simulink model "AlmostWorking_TheNotebookEdition"  (R2024b)
settings: Solver=FixedStepAuto  StartTime=0.0  StopTime=inf  RelTol=1e-3  EnableMultiTasking=on
libraries: vexarmcortexlib x20, vexcommonlib x2
settings Model: Creator=ierdn  LastModifiedBy=ierdn
settings DataIOCC: LimitDataPoints=on  SignalLoggingSaveFormat=ModelDataLogs  ReturnWorkspaceOutputs=off
settings OptimizationCC: ExpressionDepthLimit=2147483647  LifeSpan=Inf  MaxStackSize=64  EfficientTunableParamExpr=on
settings DebuggingCC: UnderspecifiedInitializationDetection=Classic  MergeDetectMultiDrivingBlocksExec=none  InheritedTsInSrcMsg=none  FcnCallInpInsideContextMsg=warning  StateNameClashWarn=warning  SFUnexpectedBacktrackingDiag=warning  SFNoUnconditionalDefaultTransitionDiag=warning  SFExecutionAtInitializationDiag=none  ArithmeticOperatorsInVariantConditions=warning
settings HardwareCC: ProdBitPerPointer=32  ProdBitPerSizeT=32  ProdBitPerPtrDiffT=32  ProdLargestAtomicInteger=Long  ProdLargestAtomicFloat=Double  ProdIntDivRoundTo=Undefined  ProdWordSize=32  ProdHWDeviceType=ARM Compatible->ARM Cortex
settings ModelReferenceCC: EnableRefExpFcnMdlSchedulingChecks=on  PropagateSignalLabelsOutOfModel=off
settings SFSimCC: MATLABDynamicMemAlloc=off  CustomCodeUndefinedFunction=UseInterfaceOnly
settings RTWCC: Description=Embedded Coder  SystemTargetFile=ert.tlc  HardwareBoard=ARM Cortex-based VEX Microcontroller  TemplateMakefile=ert_default_tmf  Toolchain=GNU Tools for VEX ARM Cortex  GPUComputeCapability=3.5
settings CodeAppCC: IgnoreCustomStorageClasses=off  CustomSymbolStrType=$N$R$M  StateflowObjectComments=on  InternalIdentifier=Classic
settings ERTTargetCC: CodeReplacementLibrary=GCC ARM Cortex-M3  MultiwordLength=2048  InlinedParameterPlacement=Hierarchical  ConvertIfToSwitch=off  SuppressUnreachableDefaultCases=off  DynamicArrayContainerType=coder::array

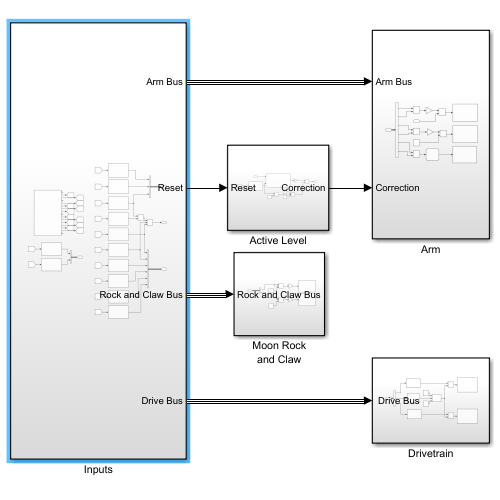
[thumbnail: Simulink's stored preview of the top-level diagram]
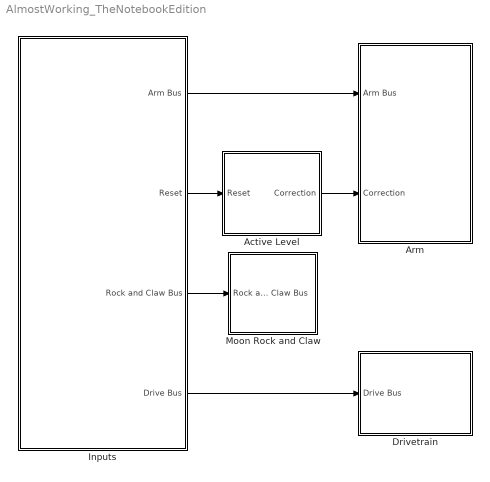
== system AlmostWorking_TheNotebookEdition ==
  Active Level : Subsystem
  Arm : Subsystem
  Drivetrain : Subsystem
  Inputs : Subsystem
  Moon Rock and Claw : Subsystem
  wires:
  Inputs/1(Arm Bus) -> Arm/1(Arm Bus)
  Inputs/3(Rock and Claw Bus) -> Moon Rock and Claw/1(Rock and Claw Bus)
  Inputs/2(Reset) -> Active Level/1(Reset)
  Inputs/4(" Drive Bus") -> Drivetrain/1(" Drive Bus")
  Active Level/1(Correction) -> Arm/2(Correction)

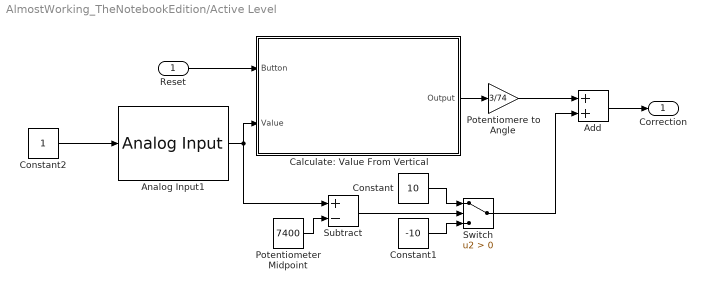
== system AlmostWorking_TheNotebookEdition/Active Level ==
  Reset : Inport
  Add : Sum
  Analog Input1 : vexarmcortexlib/Sensors/Analog Input  inChan=1  SimulationIn=on  SampleTime=0.02
  Calculate: Value From Vertical : Stateflow chart  TreatAsAtomicUnit=on
  Constant : Constant  Value=10
  Constant1 : Constant  Value=-10
  Constant2 : Constant
  Potentiomere to Angle : Gain  Gain=3/74
  Potentiometer Midpoint : Constant  Value=7400
  Subtract : Sum  Inputs=+-
  Switch : Switch  Criteria=u2 > Threshold  SaturateOnIntegerOverflow=off  InputSameDT=off
  Correction : Outport
  wires:
  Calculate: Value From Vertical/1(Output) -> Potentiomere to Angle/1
  Analog Input1/1 -> Subtract/1, Calculate: Value From Vertical/2(Value)
  Reset/1 -> Calculate: Value From Vertical/1(Button)
  Constant/1 -> Switch/1
  Constant1/1 -> Switch/3
  Potentiomere to Angle/1 -> Add/1
  Switch/1 -> Add/2
  Add/1 -> Correction/1
  Constant2/1 -> Analog Input1/1
  Subtract/1 -> Switch/2
  Potentiometer Midpoint/1 -> Subtract/2

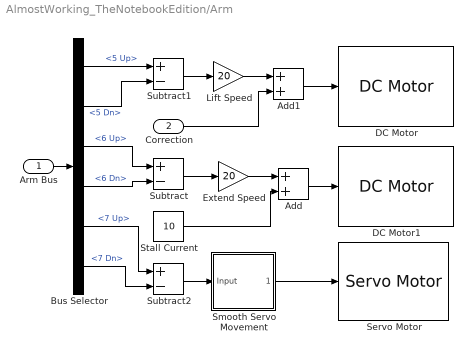
== system AlmostWorking_TheNotebookEdition/Arm ==
  Arm Bus : Inport
  Correction : Inport  Port=2
  Add : Sum
  Add1 : Sum
  Bus Selector : BusSelector  OutputSignals=5 Up,5 Dn,6 Up,6 Dn,7 Up,7 Dn
  DC Motor : vexarmcortexlib/Actuators/DC Motor  motor=8  scaleFactor=1/13.5  SimulationOut=off
  DC Motor1 : vexarmcortexlib/Actuators/DC Motor  motor=4  scaleFactor=1/13.5  SimulationOut=off
  Extend Speed : Gain  Gain=20
  Lift Speed : Gain  Gain=20
  Servo Motor : vexarmcortexlib/Actuators/Servo Motor  motor=5  scaleFactor=60/127  SimulationOut=off
  Smooth Servo Movement : Stateflow chart  TreatAsAtomicUnit=on
  Stall Current : Constant  Value=10
  Subtract : Sum  Inputs=+-
  Subtract1 : Sum  Inputs=+-
  Subtract2 : Sum  Inputs=+-
  wires:
  Bus Selector/1 -> Subtract1/1  "<5 Up>"
  Lift Speed/1 -> Add1/1
  Add1/1 -> DC Motor/1
  Stall Current/1 -> Add/2
  Subtract1/1 -> Lift Speed/1
  Bus Selector/2 -> Subtract1/2  "<5 Dn>"
  Add/1 -> DC Motor1/1
  Bus Selector/4 -> Subtract/2  "<6 Dn>"
  Subtract/1 -> Extend Speed/1
  Extend Speed/1 -> Add/1
  Bus Selector/3 -> Subtract/1  "<6 Up>"
  Bus Selector/5 -> Subtract2/1  "<7 Up>"
  Bus Selector/6 -> Subtract2/2  "<7 Dn>"
  Subtract2/1 -> Smooth Servo Movement/1(Input)
  Smooth Servo Movement/1(Output) -> Servo Motor/1
  Arm Bus/1 -> Bus Selector/1
  Correction/1 -> Add1/2

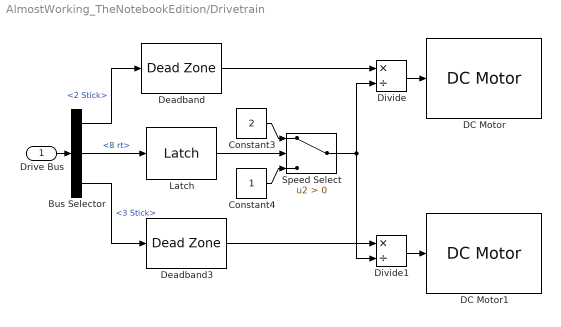
== system AlmostWorking_TheNotebookEdition/Drivetrain ==
  " Drive Bus" : Inport
  Bus Selector : BusSelector  OutputSignals=2 Stick,8 rt,3 Stick
  Constant3 : Constant  Value=2
  Constant4 : Constant
  DC Motor : vexarmcortexlib/Actuators/DC Motor  motor=2  scaleFactor=1/13.5  SimulationOut=off
  DC Motor1 : vexarmcortexlib/Actuators/DC Motor  motor=9  scaleFactor=1/13.5  SimulationOut=off
  Deadband : DeadZone  LowerValue=-9  UpperValue=9
  Deadband3 : DeadZone  LowerValue=-9  UpperValue=9
  Divide : Product  Inputs=*/
  Divide1 : Product  Inputs=*/
  Latch : vexcommonlib/Latch  output0=off  BlockPlatform=vexarmcortex
  Speed Select : Switch  Criteria=u2 > Threshold  SaturateOnIntegerOverflow=off  InputSameDT=off
  wires:
  Speed Select/1 -> Divide1/2, Divide/2
  Latch/1 -> Speed Select/2
  Constant3/1 -> Speed Select/1
  Deadband3/1 -> Divide1/1
  Constant4/1 -> Speed Select/3
  Deadband/1 -> Divide/1
  Divide/1 -> DC Motor/1
  Divide1/1 -> DC Motor1/1
  " Drive Bus"/1 -> Bus Selector/1
  Bus Selector/1 -> Deadband/1  "<2 Stick>"
  Bus Selector/3 -> Deadband3/1  "<3 Stick>"
  Bus Selector/2 -> Latch/1  "<8 rt>"

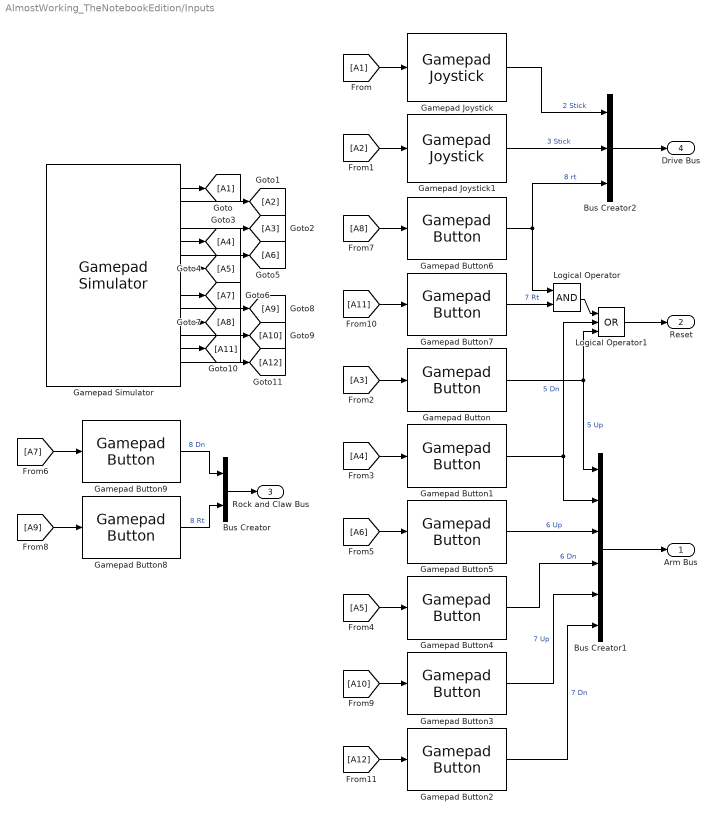
== system AlmostWorking_TheNotebookEdition/Inputs ==
  Bus Creator : BusCreator  Inputs=2
  Bus Creator1 : BusCreator  Inputs=6
  Bus Creator2 : BusCreator  Inputs=3
  Gamepad Button : vexarmcortexlib/Gamepad/Gamepad Button  joystick=1  chan=5  button56=Up  button78=Down  SimulationIn=on  SampleTime=0.02
  Gamepad Button1 : vexarmcortexlib/Gamepad/Gamepad Button  joystick=1  chan=5  button56=Down  button78=Down  SimulationIn=on  SampleTime=0.02
  Gamepad Button2 : vexarmcortexlib/Gamepad/Gamepad Button  joystick=1  chan=7  button56=Up  button78=Down  SimulationIn=on  SampleTime=0.02
  Gamepad Button3 : vexarmcortexlib/Gamepad/Gamepad Button  joystick=1  chan=7  button56=Up  button78=Up  SimulationIn=on  SampleTime=0.02
  Gamepad Button4 : vexarmcortexlib/Gamepad/Gamepad Button  joystick=1  chan=6  button56=Down  button78=Down  SimulationIn=on  SampleTime=0.02
  Gamepad Button5 : vexarmcortexlib/Gamepad/Gamepad Button  joystick=1  chan=6  button56=Up  button78=Down  SimulationIn=on  SampleTime=0.02
  Gamepad Button6 : vexarmcortexlib/Gamepad/Gamepad Button  joystick=1  chan=8  button56=Up  button78=Left  SimulationIn=on  SampleTime=0.02
  Gamepad Button7 : vexarmcortexlib/Gamepad/Gamepad Button  joystick=1  chan=7  button56=Up  button78=Right  SimulationIn=on  SampleTime=0.02
  Gamepad Button8 : vexarmcortexlib/Gamepad/Gamepad Button  joystick=1  chan=8  button56=Up  button78=Right  SimulationIn=on  SampleTime=0.02
  Gamepad Button9 : vexarmcortexlib/Gamepad/Gamepad Button  joystick=1  chan=8  button56=Up  button78=Down  SimulationIn=on  SampleTime=0.02
  Gamepad Joystick : vexarmcortexlib/Gamepad/Gamepad Joystick  joystick=1  chan=2  SimulationIn=on  SampleTime=0.02
  Gamepad Joystick1 : vexarmcortexlib/Gamepad/Gamepad Joystick  joystick=1  chan=3  SimulationIn=on  SampleTime=0.02
  Gamepad Simulator : vexcommonlib/Gamepad Simulator  WhichPad=Logitech Gamepad  JoyId=1  BlockPlatform=vexarmcortex
      settings: LibrarySourceBlock=vexarmcortexlib/Utilities/Gamepad Simulator
  Logical Operator : Logic  AllPortsSameDT=off  OutDataTypeStr=boolean
  Logical Operator1 : Logic  Operator=OR  Inputs=3  AllPortsSameDT=off  OutDataTypeStr=boolean
  Arm Bus : Outport
  Reset : Outport  Port=2
  Rock and Claw Bus : Outport  Port=3
  " Drive Bus" : Outport  Port=4
  wires:
  Gamepad Button4/1 -> Bus Creator1/4  "6 Dn"
  Gamepad Button/1 -> Logical Operator1/3, Bus Creator1/1  "5 Up"
  Gamepad Button5/1 -> Bus Creator1/3  "6 Up"
  Gamepad Button2/1 -> Bus Creator1/6  "7 Dn"
  Gamepad Joystick/1 -> Bus Creator2/1  "2 Stick"
  Gamepad Button3/1 -> Bus Creator1/5  "7 Up"
  Gamepad Joystick1/1 -> Bus Creator2/2  "3 Stick"
  Gamepad Button1/1 -> Logical Operator1/2, Bus Creator1/2  "5 Dn"
  Gamepad Button9/1 -> Bus Creator/1  "8 Dn"
  Gamepad Button8/1 -> Bus Creator/2  "8 Rt"
  Gamepad Button6/1 -> Logical Operator/1, Bus Creator2/3  "8 rt"
  Gamepad Button7/1 -> Logical Operator/2  "7 Rt"
  Bus Creator2/1 -> " Drive Bus"/1
  Logical Operator/1 -> Logical Operator1/1
  Bus Creator1/1 -> Arm Bus/1
  Bus Creator/1 -> Rock and Claw Bus/1
  Logical Operator1/1 -> Reset/1
  Gamepad Simulator/2 -> [A1]
  [A1] -> Gamepad Joystick/1
  Gamepad Simulator/3 -> [A2]
  [A2] -> Gamepad Joystick1/1
  Gamepad Simulator/5 -> [A3]
  [A3] -> Gamepad Button/1
  Gamepad Simulator/6 -> [A4]
  [A4] -> Gamepad Button1/1
  Gamepad Simulator/8 -> [A5]
  [A5] -> Gamepad Button4/1
  Gamepad Simulator/7 -> [A6]
  [A6] -> Gamepad Button5/1
  Gamepad Simulator/10 -> [A7]
  [A7] -> Gamepad Button9/1
  Gamepad Simulator/12 -> [A8]
  [A8] -> Gamepad Button6/1
  Gamepad Simulator/11 -> [A9]
  [A9] -> Gamepad Button8/1
  Gamepad Simulator/13 -> [A10]
  [A10] -> Gamepad Button3/1
  Gamepad Simulator/14 -> [A11]
  [A11] -> Gamepad Button7/1
  Gamepad Simulator/15 -> [A12]
  [A12] -> Gamepad Button2/1

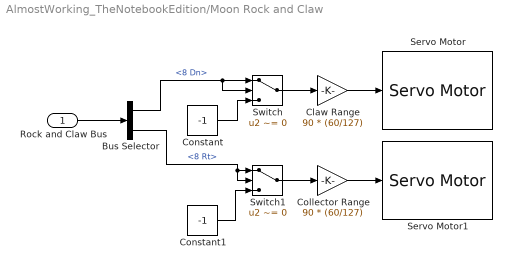
== system AlmostWorking_TheNotebookEdition/Moon Rock and Claw ==
  Rock and Claw Bus : Inport
  Bus Selector : BusSelector  OutputSignals=8 Dn,8 Rt
  Claw Range : Gain  Gain=90 * (60/127)
  Collector Range : Gain  Gain=90 * (60/127)
  Constant : Constant  Value=-1
  Constant1 : Constant  Value=-1
  Servo Motor : vexarmcortexlib/Actuators/Servo Motor  motor=6  scaleFactor=60/127  SimulationOut=off
  Servo Motor1 : vexarmcortexlib/Actuators/Servo Motor  motor=7  scaleFactor=60/127  SimulationOut=off
  Switch : Switch  Criteria=u2 ~= 0  SaturateOnIntegerOverflow=off  InputSameDT=off
  Switch1 : Switch  Criteria=u2 ~= 0  SaturateOnIntegerOverflow=off  InputSameDT=off
  wires:
  Switch1/1 -> Collector Range/1
  Bus Selector/2 -> Switch1/2, Switch1/1  "<8 Rt>"
  Collector Range/1 -> Servo Motor1/1
  Constant1/1 -> Switch1/3
  Claw Range/1 -> Servo Motor/1
  Switch/1 -> Claw Range/1
  Constant/1 -> Switch/3
  Rock and Claw Bus/1 -> Bus Selector/1
  Bus Selector/1 -> Switch/2, Switch/1  "<8 Dn>"

== stateflow chart AlmostWorking_TheNotebookEdition/Active Level/Calculate: Value From Vertical ==
  state Calculate
    Output = Value - Stored;
  state Start
    Stored = Value;
    Output = 0;
  (default) -> Start
  Start -> Calculate : [Button == 0]
  Calculate -> Start : [Button == 1]
  data: Output output; Stored local; Button input; Value input

== stateflow chart AlmostWorking_TheNotebookEdition/Arm/Smooth Servo Movement ==
  state Constant
    Speed = 0.5;
  state Change
    Output=Output+(Input*Speed);
  (default) -> Constant : {Output = 0}
  Constant -> Change : [(Input ~= 0)&&(Output >= -127 || Input == 1)&&(Output <= 127 || Input == -1)]
  Change -> Constant
  data: Input input; Output output; Speed local
